simulink model "sfcndemo_timestwo_for"  (Simulink 6.0)
settings: Solver=ode1  StartTime=0.0  StopTime=10.0  FixedStep=0.1  RelTol=1e-3
settings Model: CovMetricSettings=d  Creator=The MathWorks Inc.  LastModifiedBy=batserve  ExtModeAutoUpdateStatusClock=off
settings OptimizationCC: BlockReduction=off  BooleanDataType=off
settings DebuggingCC: CheckExecutionContextPreStartOutputMsg=on  CheckExecutionContextRuntimeOutputMsg=on  SolverPrmCheckMsg=none
settings HardwareCC: TargetUnknown=on

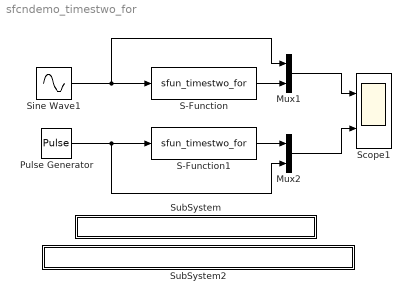
== system sfcndemo_timestwo_for ==
  Mux1 : Mux  Inputs=2
  Mux2 : Mux  Inputs=2
  Pulse Generator : DiscretePulseGenerator  PulseType=Time based  Amplitude=2  Period=1  PulseWidth=50
  S-Function : S-Function  FunctionName=sfun_timestwo_for
  S-Function1 : S-Function  FunctionName=sfun_timestwo_for
  Scope1 : Scope  NumInputPorts=2
      settings: TimeRange=10  YMin=-8~-1  YMax=8~5
  Sine Wave1 : Sin  Amplitude=3  SampleTime=0
  SubSystem : Subsystem  PropExecContextAcrossSSBoundary=on
      settings: OpenFcn=edit(fullfile(matlabroot,'simulink','src','sfun_timestwo_for.F'))
      mask Display: disp('matlabroot\simulink\src\sfun_timestwo_for.f');
  SubSystem2 : Subsystem  PropExecContextAcrossSSBoundary=on
      settings: OpenFcn=edit(fullfile(matlabroot,'toolbox','simulink','blocks','tlc_c','timestwo.tlc'))
      mask Display: disp('matlabroot\toolbox\simulink\blocks\tlc_c\sfun_timestwo_for.tlc');
  wires:
  Pulse Generator/1 -> S-Function1/1, Mux2/2
  Sine Wave1/1 -> S-Function/1, Mux1/1
  S-Function/1 -> Mux1/2
  S-Function1/1 -> Mux2/1
  Mux1/1 -> Scope1/1
  Mux2/1 -> Scope1/2

== system sfcndemo_timestwo_for/SubSystem ==

== system sfcndemo_timestwo_for/SubSystem2 ==
